simulink model "P1"  (R2018a)
settings: Solver=VariableStepAuto  StartTime=0.0  StopTime=50.0  RelTol=1e-3
settings Model: Creator=Erfan Panahi  LastModifiedBy=Erfan Panahi

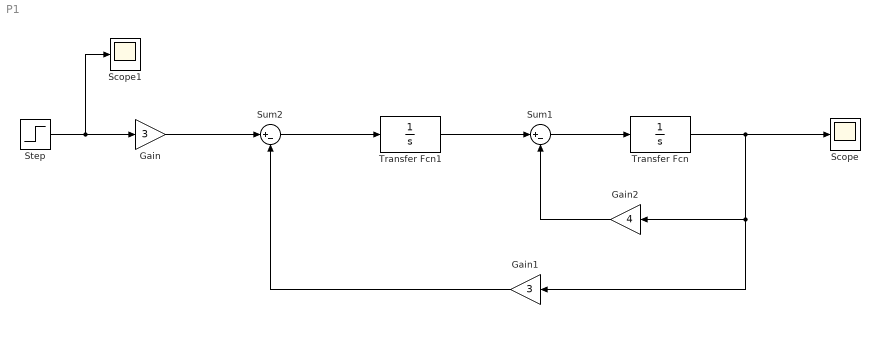
== system P1 ==
  Gain : Gain  Gain=3
  Gain1 : Gain  Gain=3
  Gain2 : Gain  Gain=4
  Scope : Scope
  Scope1 : Scope
  Step : Step  Time=0  SampleTime=0
  Sum1 : Sum  Inputs=|+-
  Sum2 : Sum  Inputs=|+-
  Transfer Fcn : TransferFcn  Denominator=[1 0]
  Transfer Fcn1 : TransferFcn  Denominator=[1 0]
  wires:
  Step/1 -> Scope1/1, Gain/1
  Gain/1 -> Sum2/1
  Sum2/1 -> Transfer Fcn1/1
  Transfer Fcn/1 -> Gain1/1, Gain2/1, Scope/1
  Gain2/1 -> Sum1/2
  Gain1/1 -> Sum2/2
  Transfer Fcn1/1 -> Sum1/1
  Sum1/1 -> Transfer Fcn/1
